simulink model "test_idealCylinder"  (R2013a)
settings: Solver=ode15s  StartTime=0.0  StopTime=5  RelTol=1e-5
libraries: fl_lib x11, nesl_utility x4, simulink x1, usask_hyd_lib x1
settings Model: Creator=tkw954  LastModifiedBy=tkw954
settings SimscapeCC: SimscapeLogType=all  SimscapeLogLimitData=off

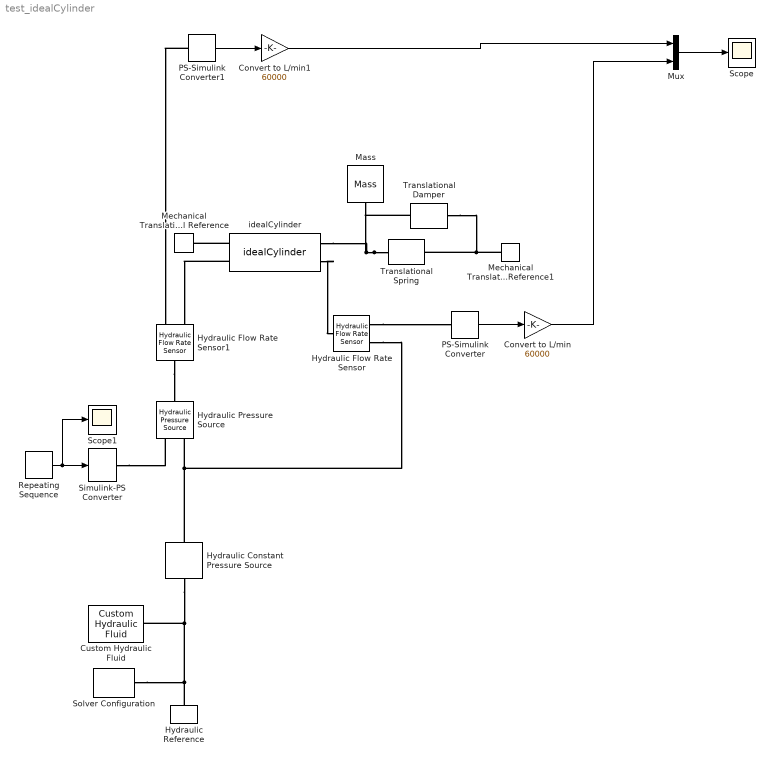
== system test_idealCylinder ==
  Convert to L/min : Gain  Gain=60000
  Convert to L/min1 : Gain  Gain=60000
  Custom Hydraulic Fluid : fl_lib/Hydraulic/Hydraulic Utilities/Custom Hydraulic Fluid  density=850 kg/m^3  viscosity_kin=18e-6 m^2/s  bulk=0.8e9 Pa  alpha=0.005  LocalVarLogging=[]
  Hydraulic Constant Pressure Source : fl_lib/Hydraulic/Hydraulic Sources/Hydraulic Constant Pressure Source  commanded_pressure=0 Pa  pressure_Log=off  flow_rate_Log=off  power_Log=off  LocalVarNames=|pressure|flow_rate|power  LocalVarDescs=|Pressure differential|Flow rate|Power generated by the source  LocalVarLogging=[0 0 0]
  Hydraulic Flow Rate Sensor : fl_lib/Hydraulic/Hydraulic Sensors/Hydraulic Flow Rate Sensor  q_Log=off  p_Log=off  LocalVarNames=|q|p  LocalVarDescs=|q|p  LocalVarLogging=[0 0]
  Hydraulic Flow Rate Sensor1 : fl_lib/Hydraulic/Hydraulic Sensors/Hydraulic Flow Rate Sensor  q_Log=off  p_Log=off  LocalVarNames=|q|p  LocalVarDescs=|q|p  LocalVarLogging=[0 0]
  Hydraulic Pressure Source : fl_lib/Hydraulic/Hydraulic Sources/Hydraulic Pressure Source  q_Log=off  p_Log=off  LocalVarNames=|q|p  LocalVarDescs=|q|p  LocalVarLogging=[0 0]
  Hydraulic Reference : fl_lib/Hydraulic/Hydraulic Elements/Hydraulic Reference  q_Log=off  LocalVarNames=|q  LocalVarDescs=|q  LocalVarLogging=0
  Mass : fl_lib/Mechanical/Translational Elements/Mass  mass=1000 kg  initial_velocity=0 m/s  f_Log=off  LocalVarNames=|f  LocalVarDescs=|f  LocalVarLogging=0
  Mechanical Translational Reference : fl_lib/Mechanical/Translational Elements/Mechanical Translational Reference  f_Log=off  LocalVarNames=|f  LocalVarDescs=|f  LocalVarLogging=0
  Mechanical Translational Reference1 : fl_lib/Mechanical/Translational Elements/Mechanical Translational Reference  f_Log=off  LocalVarNames=|f  LocalVarDescs=|f  LocalVarLogging=0
  Mux : Mux  Inputs=2
  PS-Simulink Converter : nesl_utility/PS-Simulink Converter  PhysicalDomain=network_engine_domain  SubClassName=ps_output  LeftPortType=input  RightPortType=output  PseudoPeriodic=off  Frequencies=[]  Unit=1  AffineConversion=off
  PS-Simulink Converter1 : nesl_utility/PS-Simulink Converter  PhysicalDomain=network_engine_domain  SubClassName=ps_output  LeftPortType=input  RightPortType=output  PseudoPeriodic=off  Frequencies=[]  Unit=1  AffineConversion=off
  Repeating Sequence : simulink/Sources/Repeating Sequence  rep_seq_t=[0 1 1.2 2 2.1 3 3.1 4 4.1 5]  rep_seq_y=[0 0 1 1 0 0 -1 -1 0 0]*40e6
  Scope : Scope
  Scope1 : Scope
  Simulink-PS Converter : nesl_utility/Simulink-PS Converter  PhysicalDomain=network_engine_domain  SubClassName=ps_input  LeftPortType=input  RightPortType=output  PseudoPeriodic=off  Frequencies=[]  NoiseDistribution=none  NoiseParameters=[]  Unit=1  AffineConversion=off  InputFiltering=off  SimscapeFilterOrder=1  InputFilterTimeConstant=0.001  UdotUserProvided=1
  Solver Configuration : nesl_utility/Solver Configuration  PhysicalDomain=network_engine_domain  SubClassName=solver  LeftPortType=input  RightPortType=generic  Accelerate=off  Tones=[]  Harmonics=[]  SimulateNoise=off  Profile=off  UseLocalSampling=off  EnableSwitchedLinearOptims=on  FrequencyDomain=off  UseCCode=off  UseNewInitialization=off  DoDC=off  ResidualTolerance=1e-09  UseLocalSolver=off  LocalSolverChoice=NE_BACKWARD_EULER_ADVANCER  LocalSolverSampleTime=0.001  DoFixedCost=off  MaxNonlinIter=3  MaxModeIter=2  LinearAlgebra=Sparse  DelaysMemoryBudget=1024
  Translational Damper : fl_lib/Mechanical/Translational Elements/Translational Damper  D=500e3 N/(m/s)  f_Log=off  v_Log=off  LocalVarNames=|f|v  LocalVarDescs=|f|v  LocalVarLogging=[0 0]
  Translational Spring : fl_lib/Mechanical/Translational Elements/Translational Spring  spr_rate=1e6 N/m  init_def=0 m  f_Log=off  v_Log=off  x_Log=off  LocalVarNames=|f|v|x  LocalVarDescs=|f|v|x  LocalVarLogging=[0 0 0]
  idealCylinder : usask_hyd_lib/idealCylinder  A_A=pi/4*100e-3^2  A_B=pi/4*(100e-3^2-50e-3^2)  x_min=1  dx_max=0.5  x0=1.25  K=3e8  B=1e7
  wires:
  PS-Simulink Converter/1 -> Convert to L/min/1
  PS-Simulink Converter1/1 -> Convert to L/min1/1
  Convert to L/min1/1 -> Mux/1
  Convert to L/min/1 -> Mux/2
  Mux/1 -> Scope/1
  Repeating Sequence/1 -> Scope1/1, Simulink-PS Converter/1
  connections:
  Hydraulic Reference/LConn1 -- Solver Configuration/RConn1 -- Hydraulic Constant Pressure Source/RConn1 -- Custom Hydraulic Fluid/RConn1
  Simulink-PS Converter/RConn1 -- Hydraulic Pressure Source/RConn1
  idealCylinder/RConn2 -- Hydraulic Flow Rate Sensor/LConn1
  Hydraulic Flow Rate Sensor/RConn1 -- PS-Simulink Converter/LConn1
  Hydraulic Flow Rate Sensor/RConn2 -- Hydraulic Pressure Source/RConn2 -- Hydraulic Constant Pressure Source/LConn1
  Hydraulic Flow Rate Sensor1/LConn1 -- Hydraulic Pressure Source/LConn1
  idealCylinder/LConn2 -- Hydraulic Flow Rate Sensor1/RConn2
  PS-Simulink Converter1/LConn1 -- Hydraulic Flow Rate Sensor1/RConn1
  idealCylinder/LConn1 -- Mechanical Translational Reference/LConn1
  Translational Spring/LConn1 -- idealCylinder/RConn1 -- Translational Damper/LConn1 -- Mass/LConn1
  Mechanical Translational Reference1/LConn1 -- Translational Damper/RConn1 -- Translational Spring/RConn1
